simulink model "SA_chirp_modified"  (Simulink 9.2)
settings: Solver=FixedStepDiscrete  StartTime=0.0  StopTime=100  RelTol=1e-3
libraries: dspsigops x2, simulink x1, dsparch4 x1, dspspect3 x1
settings Model: Creator=DSPadmin  LastModifiedBy=mawil
settings DataIOCC: SaveOutput=off  SignalLogging=off  SaveTime=off
settings OptimizationCC: DefaultParameterBehavior=Inlined  RollThreshold=2  InitFltsAndDblsToZero=on
settings DebuggingCC: AlgebraicLoopMsg=error  SaveWithParameterizedLinksMsg=none  SignalResolutionControl=TryResolveAllWithWarning  SolverPrmCheckMsg=warning  MultiTaskDSMMsg=warning  MultiTaskCondExecSysMsg=none  SingleTaskRateTransMsg=error  StateNameClashWarn=none
settings GRTTargetCC: TargetFcnLib=ansi_tfl_tmw.mat

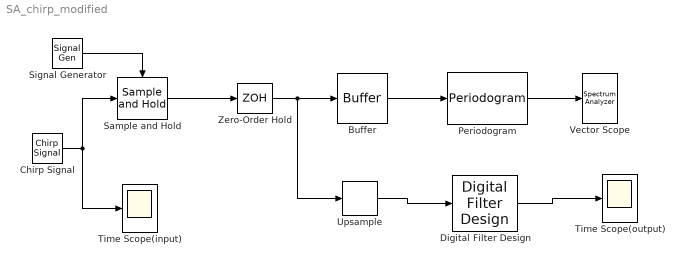
== system SA_chirp_modified ==
  Buffer : Buffer  N=256
  Chirp Signal : simulink/Sources/Chirp Signal  f1=10  T=100  f2=900
  Digital Filter Design : dsparch4/Digital Filter Design  mwdsp_browser_bugfix_var=off
  Periodogram : dspspect3/Periodogram  measurement=Power spectral density  wintype=Hamming  Rs=50  beta=5  winsamp=Symmetric  FFTImplementation=Auto  inheritFFT=off  fftsize=256  navg=4  inheritTs=on  Ts=1
      settings: SourceProductName=DSP System Toolbox  SourceProductBaseCode=DS
  Sample and Hold : dspsigops/Sample and Hold  trig=Rising edge  initCond=0  latchinput=off
  Signal Generator : SignalGenerator  WaveForm=square  Frequency=1000
  Time Scope(input) : Scope
  Time Scope(output) : Scope
  Upsample : dspsigops/Upsample  N=8  phase=0  InputProcessing=Columns as channels (frame based)  RateOptions=Allow multirate processing  ic=0  mode=Unused parameter value
  "Vector Scope " : SpectrumAnalyzer
  Zero-Order Hold : ZeroOrderHold  SampleTime=1/1000
  wires:
  Signal Generator/1 -> Sample and Hold/Trigger
  Chirp Signal/1 -> Sample and Hold/1, Time Scope(input)/1
  Sample and Hold/1 -> Zero-Order Hold/1
  Zero-Order Hold/1 -> Buffer/1, Upsample/1
  Buffer/1 -> Periodogram/1
  Upsample/1 -> Digital Filter Design/1
  Digital Filter Design/1 -> Time Scope(output)/1
  Periodogram/1 -> "Vector Scope "/1
